simulink subsystem "time_ctrl"  (R2021b)
settings: Solver=VariableStepAuto  StartTime=0.0  StopTime=10.0  RelTol=1e-3
undefined symbols (not defined in the file): frame_size, symbol_size, ts_bitwidth
libraries: simulink x1
settings Model: Creator=torha  LastModifiedBy=torha
settings SolverCC: AlgebraicLoopSolver=TrustRegion
settings DebuggingCC: SFMachineParentedDataDiag=warning

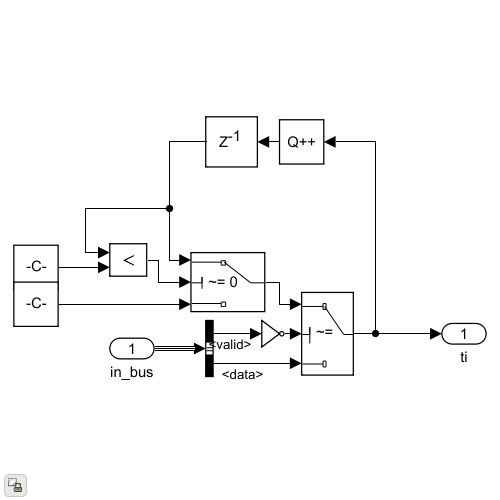
[thumbnail: Simulink's stored preview of the top-level diagram]
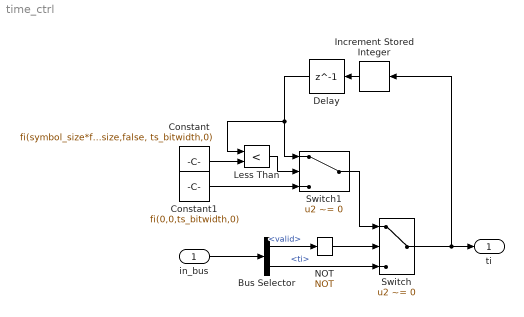
== system time_ctrl ==
  in_bus : Inport
  Bus Selector : BusSelector  OutputSignals=valid,ti
  Constant : Constant  Value=fi(symbol_size*frame_size,false, ts_bitwidth,0)
  Constant1 : Constant  Value=fi(0,0,ts_bitwidth,0)
  Delay : Delay  DelayLength=1  InitialCondition=fi(1, 0, ts_bitwidth, 0)
  Increment Stored Integer : simulink/Additional Math & Discrete/Additional Math: Increment - Decrement/Increment Stored Integer
  Less Than : RelationalOperator  Operator=<  OutDataTypeStr=boolean  RndMeth=Simplest
  NOT : Logic  Operator=NOT  IconShape=distinctive  AllPortsSameDT=off  OutDataTypeStr=boolean
  Switch : Switch  Criteria=u2 ~= 0
  Switch1 : Switch  Criteria=u2 ~= 0
  ti : Outport
  wires:
  Switch/1 -> ti/1, Increment Stored Integer/1
  in_bus/1 -> Bus Selector/1
  Bus Selector/1 -> NOT/1  "<valid>"
  Bus Selector/2 -> Switch/3  "<ti>"
  Switch1/1 -> Switch/1
  Delay/1 -> Less Than/1, Switch1/1
  Less Than/1 -> Switch1/2
  Constant/1 -> Less Than/2
  Constant1/1 -> Switch1/3
  NOT/1 -> Switch/2
  Increment Stored Integer/1 -> Delay/1
